simulink model "IEEE14_case"  (R2024b)
settings: Solver=FixedStepAuto  StartTime=0  StopTime=2  FixedStep=1e-7  RelTol=1e-3
values from neighbouring files (symbols this model uses):
  GFL_15_Bva = 0.009    [IEEE14_parameters.m]
  GFL_15_C_bus_pu = 7.179419    [IEEE14_parameters.m]
  GFL_15_f0 = 60    [IEEE14_parameters.m]
  GFL_15_I_id = 691.26967    [IEEE14_parameters.m]
  GFL_15_I_iq = 691.26967    [IEEE14_parameters.m]
  GFL_15_I_od = 45.2207    [IEEE14_parameters.m]
  GFL_15_I_oq = 45.2207    [IEEE14_parameters.m]
  GFL_15_I_pll = 0.78    [IEEE14_parameters.m]
  GFL_15_Kdi = 0.09    [IEEE14_parameters.m]
  GFL_15_Kdo = 0.9    [IEEE14_parameters.m]
  GFL_15_Kqi = 0.09    [IEEE14_parameters.m]
  GFL_15_Kqo = 0.9    [IEEE14_parameters.m]
  GFL_15_Lg_pu = 0.631447    [IEEE14_parameters.m]
  GFL_15_mode = 1    [IEEE14_parameters.m]
  GFL_15_P_id = 3.7166    [IEEE14_parameters.m]
  GFL_15_P_iq = 3.7166    [IEEE14_parameters.m]
  GFL_15_P_od = 0.4798    [IEEE14_parameters.m]
  GFL_15_P_oq = 0.4798    [IEEE14_parameters.m]
  GFL_15_P_pll = 290.42    [IEEE14_parameters.m]
  GFL_15_Qe_ref = 0.2    [IEEE14_parameters.m]
  GFL_15_Rg_pu = 0.024016    [IEEE14_parameters.m]
  GFL_15_Sbase = 1.000000e+4    (= 10000)    [IEEE14_parameters.m]
  GFL_15_Tdi = 0.01    [IEEE14_parameters.m]
  GFL_15_Tdo = 0.2    [IEEE14_parameters.m]
  GFL_15_Tqi = 0.01    [IEEE14_parameters.m]
  GFL_15_Tqo = 0.2    [IEEE14_parameters.m]
  GFL_15_Vbase = 380    [IEEE14_parameters.m]
  GFL_15_Vdc_ref = 1.011475    [IEEE14_parameters.m]
  GFL_15_Vdcbase = 700    [IEEE14_parameters.m]
  GFL_15_vq_ref = 0    [IEEE14_parameters.m]
  GFL_16_Bva = 0.002    [IEEE14_parameters.m]
  GFL_16_C_bus_pu = 7.179419    [IEEE14_parameters.m]
  GFL_16_f0 = 60    [IEEE14_parameters.m]
  GFL_16_I_id = 691.26967    [IEEE14_parameters.m]
  GFL_16_I_iq = 691.26967    [IEEE14_parameters.m]
  GFL_16_I_od = 45.2207    [IEEE14_parameters.m]
  GFL_16_I_oq = 45.2207    [IEEE14_parameters.m]
  GFL_16_I_pll = 0.78    [IEEE14_parameters.m]
  GFL_16_Kdi = 0.05    [IEEE14_parameters.m]
  GFL_16_Kdo = 0.5    [IEEE14_parameters.m]
  GFL_16_Kqi = 0.05    [IEEE14_parameters.m]
  GFL_16_Kqo = 0.5    [IEEE14_parameters.m]
  GFL_16_Lg_pu = 0.631447    [IEEE14_parameters.m]
  GFL_16_mode = 1    [IEEE14_parameters.m]
  GFL_16_P_id = 3.7166    [IEEE14_parameters.m]
  GFL_16_P_iq = 3.7166    [IEEE14_parameters.m]
  GFL_16_P_od = 0.4798    [IEEE14_parameters.m]
  GFL_16_P_oq = 0.4798    [IEEE14_parameters.m]
  GFL_16_P_pll = 290.42    [IEEE14_parameters.m]
  GFL_16_Qe_ref = 0.2    [IEEE14_parameters.m]
  GFL_16_Rg_pu = 0.024016    [IEEE14_parameters.m]
  GFL_16_Sbase = 1.000000e+4    (= 10000)    [IEEE14_parameters.m]
  GFL_16_Tdi = 0.01    [IEEE14_parameters.m]
  GFL_16_Tdo = 0.2    [IEEE14_parameters.m]
  GFL_16_Tqi = 0.01    [IEEE14_parameters.m]
  GFL_16_Tqo = 0.2    [IEEE14_parameters.m]
  GFL_16_Vbase = 380    [IEEE14_parameters.m]
  GFL_16_Vdc_ref = 1.01144    [IEEE14_parameters.m]
  GFL_16_Vdcbase = 700    [IEEE14_parameters.m]
  GFL_16_vq_ref = 0    [IEEE14_parameters.m]
  GFL_17_Bva = 0.002    [IEEE14_parameters.m]
  GFL_17_C_bus_pu = 7.179419    [IEEE14_parameters.m]
  GFL_17_f0 = 60    [IEEE14_parameters.m]
  GFL_17_I_id = 691.26967    [IEEE14_parameters.m]
  GFL_17_I_iq = 691.26967    [IEEE14_parameters.m]
  GFL_17_I_od = 45.2207    [IEEE14_parameters.m]
  GFL_17_I_oq = 45.2207    [IEEE14_parameters.m]
  GFL_17_I_pll = 0.78    [IEEE14_parameters.m]
  GFL_17_Kdi = 0.05    [IEEE14_parameters.m]
  GFL_17_Kdo = 0.5    [IEEE14_parameters.m]
  GFL_17_Kqi = 0.05    [IEEE14_parameters.m]
  GFL_17_Kqo = 0.5    [IEEE14_parameters.m]
  GFL_17_Lg_pu = 0.631447    [IEEE14_parameters.m]
  GFL_17_mode = 1    [IEEE14_parameters.m]
  GFL_17_P_id = 3.7166    [IEEE14_parameters.m]
  GFL_17_P_iq = 3.7166    [IEEE14_parameters.m]
  GFL_17_P_od = 0.4798    [IEEE14_parameters.m]
  GFL_17_P_oq = 0.4798    [IEEE14_parameters.m]
  GFL_17_P_pll = 290.42    [IEEE14_parameters.m]
  GFL_17_Qe_ref = 0.2    [IEEE14_parameters.m]
  GFL_17_Rg_pu = 0.024016    [IEEE14_parameters.m]
  GFL_17_Sbase = 1.000000e+4    (= 10000)    [IEEE14_parameters.m]
  GFL_17_Tdi = 0.01    [IEEE14_parameters.m]
  GFL_17_Tdo = 0.2    [IEEE14_parameters.m]
  GFL_17_Tqi = 0.01    [IEEE14_parameters.m]
  GFL_17_Tqo = 0.2    [IEEE14_parameters.m]
  GFL_17_Vbase = 380    [IEEE14_parameters.m]
  GFL_17_Vdc_ref = 1.011632    [IEEE14_parameters.m]
  GFL_17_Vdcbase = 700    [IEEE14_parameters.m]
  GFL_17_vq_ref = 0    [IEEE14_parameters.m]
  GFL_18_Bva = 0.002    [IEEE14_parameters.m]
  GFL_18_C_bus_pu = 7.179419    [IEEE14_parameters.m]
  GFL_18_f0 = 60    [IEEE14_parameters.m]
  GFL_18_I_id = 691.26967    [IEEE14_parameters.m]
  GFL_18_I_iq = 691.26967    [IEEE14_parameters.m]
  GFL_18_I_od = 45.2207    [IEEE14_parameters.m]
  GFL_18_I_oq = 45.2207    [IEEE14_parameters.m]
  GFL_18_I_pll = 0.78    [IEEE14_parameters.m]
  GFL_18_Kdi = 0.05    [IEEE14_parameters.m]
  GFL_18_Kdo = 0.5    [IEEE14_parameters.m]
  GFL_18_Kqi = 0.05    [IEEE14_parameters.m]
  GFL_18_Kqo = 0.5    [IEEE14_parameters.m]
  GFL_18_Lg_pu = 0.631447    [IEEE14_parameters.m]
  GFL_18_mode = 1    [IEEE14_parameters.m]
  GFL_18_P_id = 3.7166    [IEEE14_parameters.m]
  GFL_18_P_iq = 3.7166    [IEEE14_parameters.m]
  GFL_18_P_od = 0.4798    [IEEE14_parameters.m]
  GFL_18_P_oq = 0.4798    [IEEE14_parameters.m]
  GFL_18_P_pll = 290.42    [IEEE14_parameters.m]
  GFL_18_Qe_ref = 0.2    [IEEE14_parameters.m]
  GFL_18_Rg_pu = 0.024016    [IEEE14_parameters.m]
  GFL_18_Sbase = 1.000000e+4    (= 10000)    [IEEE14_parameters.m]
  GFL_18_Tdi = 0.01    [IEEE14_parameters.m]
  GFL_18_Tdo = 0.2    [IEEE14_parameters.m]
  GFL_18_Tqi = 0.01    [IEEE14_parameters.m]
  GFL_18_Tqo = 0.2    [IEEE14_parameters.m]
  GFL_18_Vbase = 380    [IEEE14_parameters.m]
  GFL_18_Vdc_ref = 1.011572    [IEEE14_parameters.m]
  GFL_18_Vdcbase = 700    [IEEE14_parameters.m]
  GFL_18_vq_ref = 0    [IEEE14_parameters.m]
  ... (+180 more)
(part 12 of 25)

== system IEEE14_case/GFL_16/d_i_gq_GFL_16_block ==
  note: d_i_gq_GFL_16 in case14gfl
      | $\frac{2\,\pi \,\mathrm{Sbase}\,f_{0}\,\left(\Phi _{\mathrm{gd},\mathrm{GFL},16}+P_{\mathrm{iq}}\,\left(\mathrm{Iqv}_{\mathrm{GFL},16}+\Phi _{\mathrm{gc},\mathrm{GFL},16}-i_{\mathrm{gq},\mathrm{GFL},16}-P_{\mathrm{oq}}\,\left(\mathrm{Qe}_{\mathrm{ref}}\,\mathrm{Sbase}+1.73205080756888\,\mathrm{Vbase}\,i_{\mathrm{gd},\mathrm{GFL},16}\,\left(v_{q,\mathrm{GFL},16}\,\cos\left(\theta _{\mathrm{pll},\mathrm{GFL},16}\right)+v_{d,\mathrm{GFL},16}\,\sin\left(\theta _{\mathrm{pll},\mathrm{GFL},16}\right)\right)+1.73205080756888\,\mathrm{Vbase}\,i_{\mathrm{gq},\mathrm{GFL},16}\,\left(v_{d,\mathrm{GFL},16}\,\cos\left(\theta _{\mathrm{pll},\mathrm{GFL},16}\right)-v_{q,\mathrm{GFL},16}\,\sin\left(\theta _{\mathrm{pll},\mathrm{GFL},16}\right)\right)\right)+\mathrm{Bva}\,\mathrm{Vbase}\,\left(v_{q,\mathrm{GFL},16}\,\cos\left(\theta _{\mathrm{pll},\mathrm{GFL},16}\right)+v_{d,\mathrm{GFL},16}\,\sin\left(\theta _{\mathrm{pll},\mathrm{GFL},16}\right)\right)\right)-\frac{\mathrm{Rg}_{\mathrm{pu}}\,{\mathrm{Vbase}}^2\,i_{\mathrm{gq},\mathrm{GFL},16}}{\mathrm{Sbase}}\right)}{\mathrm{Lg}_{\mathrm{pu}}\,{\mathrm{Vbase}}^2}$
      | Automatically generated on 2025-10-09 21:35:48 .
  Input_v_d_GFL_16_26005 : Inport
  State_theta_pll_GFL_16_b9b0c : Inport  Port=2
  Input_v_q_GFL_16_f5e00 : Inport  Port=3
  State_theta_pll_GFL_16_3325f : Inport  Port=4
  State_Iqv_GFL_16_fce4f : Inport  Port=5
  State_i_gd_GFL_16_461cd : Inport  Port=6
  Input_v_d_GFL_16_21396 : Inport  Port=7
  State_theta_pll_GFL_16_b6938 : Inport  Port=8
  Input_v_q_GFL_16_5c00e : Inport  Port=9
  State_theta_pll_GFL_16_ce5b5 : Inport  Port=10
  State_i_gq_GFL_16_8af0d : Inport  Port=11
  Input_v_d_GFL_16_f3aaf : Inport  Port=12
  State_theta_pll_GFL_16_f68d0 : Inport  Port=13
  Input_v_q_GFL_16_4d2d7 : Inport  Port=14
  State_theta_pll_GFL_16_2ae3b : Inport  Port=15
  State_Phi_gc_GFL_16_ded18 : Inport  Port=16
  State_i_gq_GFL_16_f0d16 : Inport  Port=17
  State_Phi_gd_GFL_16_6ff49 : Inport  Port=18
  State_i_gq_GFL_16_bb299 : Inport  Port=19
  Add_1f236 : Sum
  Add_902ad : Sum
  Add_90e5e : Sum
  Add_b2698 : Sum
  Add_d010b : Sum
  Add_ed010 : Sum
  Constant_-1_4b2a3 : Constant  Value=-1
  Constant_1.73205080756888_41091 : Constant  Value=1.73205080756888
  Constant_1.73205080756888_fcb3e : Constant  Value=1.73205080756888
  Constant_2.0_22626 : Constant  Value=2.0
  Constant_2.0_38ada : Constant  Value=2.0
  Constant_2.0_a6037 : Constant  Value=2.0
  Constant_Bva_7a2f5 : Constant  Value=Bva
  Constant_Lg_pu_7f2f3 : Constant  Value=Lg_pu
  Constant_P_iq_ae706 : Constant  Value=P_iq
  Constant_P_oq_d800d : Constant  Value=P_oq
  Constant_Qe_ref_48f82 : Constant  Value=Qe_ref
  Constant_Rg_pu_1fb6c : Constant  Value=Rg_pu
  Constant_Sbase_2a5f4 : Constant  Value=Sbase
  Constant_Sbase_8d4df : Constant  Value=Sbase
  Constant_Sbase_d2429 : Constant  Value=Sbase
  Constant_Vbase_52c7c : Constant  Value=Vbase
  Constant_Vbase_77d71 : Constant  Value=Vbase
  Constant_Vbase_9d288 : Constant  Value=Vbase
  Constant_Vbase_cc3fd : Constant  Value=Vbase
  Constant_Vbase_f36e9 : Constant  Value=Vbase
  Constant_f0_15919 : Constant  Value=f0
  Constant_pi_ae5c5 : Constant  Value=pi
  Divide_358c2 : Product  Inputs=*/
  Divide_d98bc : Product  Inputs=*/
  MathFunc_cos_1f83c : Trigonometry  Operator=cos
  MathFunc_cos_2f6c0 : Trigonometry  Operator=cos
  MathFunc_cos_612b0 : Trigonometry  Operator=cos
  MathFunc_sin_4af8b : Trigonometry
  MathFunc_sin_9c669 : Trigonometry
  MathFunc_sin_cb3b8 : Trigonometry
  Power_64a0d : Math  Operator=pow
  Power_c9ffe : Math  Operator=pow
  Product_0ecab : Product
  Product_0f8e8 : Product
  Product_125e1 : Product
  Product_2253b : Product
  Product_24ac4 : Product
  Product_3d9b9 : Product
  Product_45584 : Product
  Product_5de20 : Product
  Product_630cf : Product
  Product_76e52 : Product
  Product_7ef05 : Product
  Product_7fa9f : Product
  Product_93679 : Product
  Product_95eb5 : Product
  Product_96ca3 : Product
  Product_9f0a3 : Product
  Product_a28aa : Product
  Product_a51bb : Product
  Product_c0fca : Product
  Product_d9703 : Product
  Product_e0f5e : Product
  Product_e1d29 : Product
  Product_f68a2 : Product
  Product_fdb7e : Product
  Product_ffb6f : Product
  Subtract_3c982 : Sum  Inputs=+-
  Subtract_9e73c : Sum  Inputs=+-
  Subtract_aaa71 : Sum  Inputs=+-
  Subtract_dcd4c : Sum  Inputs=+-
  Subtract_f9644 : Sum  Inputs=+-
  Blockout_d_i_gq_GFL_16_4ea9b : Outport
  wires:
  State_theta_pll_GFL_16_b6938/1 -> MathFunc_sin_9c669/1
  MathFunc_sin_9c669/1 -> Product_93679/2
  Subtract_f9644/1 -> Product_e1d29/2
  Constant_Vbase_f36e9/1 -> Product_c0fca/2
  State_theta_pll_GFL_16_ce5b5/1 -> MathFunc_cos_2f6c0/1
  MathFunc_cos_2f6c0/1 -> Product_9f0a3/2
  Product_c0fca/1 -> Product_fdb7e/1
  Constant_1.73205080756888_41091/1 -> Product_c0fca/1
  Product_93679/1 -> Add_d010b/1
  Input_v_d_GFL_16_21396/1 -> Product_93679/1
  Input_v_q_GFL_16_5c00e/1 -> Product_9f0a3/1
  Constant_Sbase_d2429/1 -> Product_5de20/2
  MathFunc_cos_612b0/1 -> Product_96ca3/2
  State_Phi_gd_GFL_16_6ff49/1 -> Add_ed010/2
  State_theta_pll_GFL_16_f68d0/1 -> MathFunc_cos_612b0/1
  Product_9f0a3/1 -> Add_d010b/2
  Constant_Sbase_8d4df/1 -> Divide_358c2/2
  State_theta_pll_GFL_16_2ae3b/1 -> MathFunc_sin_4af8b/1
  MathFunc_sin_cb3b8/1 -> Product_0f8e8/2
  State_theta_pll_GFL_16_b9b0c/1 -> MathFunc_sin_cb3b8/1
  State_theta_pll_GFL_16_3325f/1 -> MathFunc_cos_1f83c/1
  Constant_-1_4b2a3/1 -> Product_ffb6f/1
  Constant_Qe_ref_48f82/1 -> Product_ffb6f/2
  Constant_1.73205080756888_fcb3e/1 -> Product_a51bb/1
  State_i_gd_GFL_16_461cd/1 -> Product_fdb7e/2
  Constant_Vbase_52c7c/1 -> Power_c9ffe/1
  Product_3d9b9/1 -> Add_1f236/1
  Constant_Vbase_cc3fd/1 -> Product_a51bb/2
  State_i_gq_GFL_16_f0d16/1 -> Subtract_9e73c/2
  Input_v_d_GFL_16_f3aaf/1 -> Product_96ca3/1
  Input_v_q_GFL_16_4d2d7/1 -> Product_a28aa/1
  Constant_2.0_22626/1 -> Product_7ef05/1
  MathFunc_sin_4af8b/1 -> Product_a28aa/2
  Product_a28aa/1 -> Subtract_dcd4c/2
  Input_v_d_GFL_16_26005/1 -> Product_0f8e8/1
  Input_v_q_GFL_16_f5e00/1 -> Product_7fa9f/1
  Subtract_dcd4c/1 -> Product_e0f5e/2
  MathFunc_cos_1f83c/1 -> Product_7fa9f/2
  Product_ffb6f/1 -> Product_5de20/1
  Product_fdb7e/1 -> Product_d9703/1
  Add_d010b/1 -> Product_d9703/2
  Add_90e5e/1 -> Subtract_9e73c/1
  Product_a51bb/1 -> Product_630cf/1
  State_i_gq_GFL_16_8af0d/1 -> Product_630cf/2
  Product_96ca3/1 -> Subtract_dcd4c/1
  Constant_Bva_7a2f5/1 -> Product_2253b/1
  Constant_pi_ae5c5/1 -> Product_7ef05/2
  Constant_Vbase_9d288/1 -> Product_2253b/2
  Product_0f8e8/1 -> Add_902ad/1
  Product_7fa9f/1 -> Add_902ad/2
  Subtract_9e73c/1 -> Product_24ac4/2
  Product_5de20/1 -> Subtract_aaa71/1
  Constant_Vbase_77d71/1 -> Power_64a0d/1
  Product_d9703/1 -> Subtract_aaa71/2
  Product_630cf/1 -> Product_e0f5e/1
  Power_c9ffe/1 -> Product_f68a2/2
  Product_2253b/1 -> Product_3d9b9/1
  Constant_Sbase_2a5f4/1 -> Product_45584/2
  Add_902ad/1 -> Product_3d9b9/2
  Subtract_aaa71/1 -> Subtract_f9644/1
  Product_e0f5e/1 -> Subtract_f9644/2
  State_Iqv_GFL_16_fce4f/1 -> Add_1f236/2
  Constant_P_oq_d800d/1 -> Product_e1d29/1
  Add_1f236/1 -> Add_b2698/1
  Product_e1d29/1 -> Add_b2698/2
  Add_b2698/1 -> Add_90e5e/1
  State_Phi_gc_GFL_16_ded18/1 -> Add_90e5e/2
  Constant_2.0_a6037/1 -> Power_c9ffe/2
  Constant_Rg_pu_1fb6c/1 -> Product_f68a2/1
  Constant_P_iq_ae706/1 -> Product_24ac4/1
  Product_f68a2/1 -> Product_0ecab/1
  State_i_gq_GFL_16_bb299/1 -> Product_0ecab/2
  Product_7ef05/1 -> Product_45584/1
  Product_24ac4/1 -> Add_ed010/1
  Product_0ecab/1 -> Divide_358c2/1
  Product_45584/1 -> Product_76e52/1
  Constant_f0_15919/1 -> Product_76e52/2
  Add_ed010/1 -> Subtract_3c982/1
  Divide_358c2/1 -> Subtract_3c982/2
  Constant_2.0_38ada/1 -> Power_64a0d/2
  Product_76e52/1 -> Product_95eb5/1
  Subtract_3c982/1 -> Product_95eb5/2
  Constant_Lg_pu_7f2f3/1 -> Product_125e1/1
  Power_64a0d/1 -> Product_125e1/2
  Product_95eb5/1 -> Divide_d98bc/1
  Product_125e1/1 -> Divide_d98bc/2
  Divide_d98bc/1 -> Blockout_d_i_gq_GFL_16_4ea9b/1

== system IEEE14_case/GFL_16/d_theta_pll_GFL_16_block ==
  note: d_theta_pll_GFL_16 in case14gfl
      | $\mathrm{Phipll}_{\mathrm{GFL},16}-P_{\mathrm{pll}}\,\left(\mathrm{vq}_{\mathrm{ref}}+v_{q,\mathrm{GFL},16}\,\cos\left(\theta _{\mathrm{pll},\mathrm{GFL},16}\right)+v_{d,\mathrm{GFL},16}\,\sin\left(\theta _{\mathrm{pll},\mathrm{GFL},16}\right)\right)$
      | Automatically generated on 2025-10-09 21:36:05 .
  Input_v_d_GFL_16_c3931 : Inport
  State_theta_pll_GFL_16_60b13 : Inport  Port=2
  Input_v_q_GFL_16_f8c47 : Inport  Port=3
  State_theta_pll_GFL_16_eb390 : Inport  Port=4
  State_Phipll_GFL_16_9e2b9 : Inport  Port=5
  Add_7626c : Sum
  Constant_-1_d55e9 : Constant  Value=-1
  Constant_P_pll_b3652 : Constant  Value=P_pll
  Constant_vq_ref_9ec67 : Constant  Value=vq_ref
  MathFunc_cos_68f81 : Trigonometry  Operator=cos
  MathFunc_sin_003f3 : Trigonometry
  Product_2e053 : Product
  Product_35cda : Product
  Product_c0d6e : Product
  Product_c6d12 : Product
  Subtract_48f00 : Sum  Inputs=+-
  Subtract_4de10 : Sum  Inputs=+-
  Blockout_d_theta_pll_GFL_16_374a4 : Outport
  wires:
  Constant_vq_ref_9ec67/1 -> Subtract_4de10/2
  MathFunc_cos_68f81/1 -> Product_c0d6e/2
  Product_2e053/1 -> Product_c6d12/1
  Constant_-1_d55e9/1 -> Product_2e053/1
  Input_v_d_GFL_16_c3931/1 -> Product_2e053/2
  State_theta_pll_GFL_16_60b13/1 -> MathFunc_sin_003f3/1
  State_theta_pll_GFL_16_eb390/1 -> MathFunc_cos_68f81/1
  MathFunc_sin_003f3/1 -> Product_c6d12/2
  Input_v_q_GFL_16_f8c47/1 -> Product_c0d6e/1
  Product_c6d12/1 -> Subtract_48f00/1
  Product_c0d6e/1 -> Subtract_48f00/2
  Subtract_48f00/1 -> Subtract_4de10/1
  Constant_P_pll_b3652/1 -> Product_35cda/1
  Subtract_4de10/1 -> Product_35cda/2
  Product_35cda/1 -> Add_7626c/1
  State_Phipll_GFL_16_9e2b9/1 -> Add_7626c/2
  Add_7626c/1 -> Blockout_d_theta_pll_GFL_16_374a4/1

== system IEEE14_case/GFL_16/e_dc_GFL_16_block ==
  note: e_dc_GFL_16 in case14gfl
      | $\frac{V_{\mathrm{dc},\mathrm{GFL},16}}{\mathrm{Vdcbase}}$
      | Automatically generated on 2025-10-09 21:36:23 .
  State_V_dc_GFL_16_ba6ae : Inport
  Constant_Vdcbase_fd435 : Constant  Value=Vdcbase
  Divide_18da4 : Product  Inputs=*/
  Blockout_e_dc_GFL_16_30897 : Outport
  wires:
  State_V_dc_GFL_16_ba6ae/1 -> Divide_18da4/1
  Constant_Vdcbase_fd435/1 -> Divide_18da4/2
  Divide_18da4/1 -> Blockout_e_dc_GFL_16_30897/1

== system IEEE14_case/GFL_16/i_d_GFL_16_block ==
  note: i_d_GFL_16 in case14gfl
      | $0.00658179306876173\,i_{\mathrm{gd},\mathrm{GFL},16}\,\cos\left(\theta _{\mathrm{pll},\mathrm{GFL},16}\right)+0.00658179306876173\,i_{\mathrm{gq},\mathrm{GFL},16}\,\sin\left(\theta _{\mathrm{pll},\mathrm{GFL},16}\right)$
      | Automatically generated on 2025-10-09 21:36:22 .
  State_i_gd_GFL_16_f9181 : Inport
  State_theta_pll_GFL_16_be048 : Inport  Port=2
  State_i_gq_GFL_16_5d9af : Inport  Port=3
  State_theta_pll_GFL_16_4b91a : Inport  Port=4
  Add_e2555 : Sum
  Constant_0.00658179306876173_ae954 : Constant  Value=0.00658179306876173
  Constant_0.00658179306876173_b6366 : Constant  Value=0.00658179306876173
  MathFunc_cos_8767b : Trigonometry  Operator=cos
  MathFunc_sin_49c71 : Trigonometry
  Product_74789 : Product
  Product_a340e : Product
  Product_b858c : Product
  Product_e5950 : Product
  Blockout_i_d_GFL_16_cb76b : Outport
  wires:
  Constant_0.00658179306876173_ae954/1 -> Product_74789/1
  State_i_gd_GFL_16_f9181/1 -> Product_74789/2
  Constant_0.00658179306876173_b6366/1 -> Product_a340e/1
  Product_74789/1 -> Product_e5950/1
  State_theta_pll_GFL_16_be048/1 -> MathFunc_cos_8767b/1
  MathFunc_sin_49c71/1 -> Product_b858c/2
  State_theta_pll_GFL_16_4b91a/1 -> MathFunc_sin_49c71/1
  State_i_gq_GFL_16_5d9af/1 -> Product_a340e/2
  MathFunc_cos_8767b/1 -> Product_e5950/2
  Product_a340e/1 -> Product_b858c/1
  Product_e5950/1 -> Add_e2555/1
  Product_b858c/1 -> Add_e2555/2
  Add_e2555/1 -> Blockout_i_d_GFL_16_cb76b/1

== system IEEE14_case/GFL_16/i_q_GFL_16_block ==
  note: i_q_GFL_16 in case14gfl
      | $0.00658179306876173\,i_{\mathrm{gq},\mathrm{GFL},16}\,\cos\left(\theta _{\mathrm{pll},\mathrm{GFL},16}\right)-0.00658179306876173\,i_{\mathrm{gd},\mathrm{GFL},16}\,\sin\left(\theta _{\mathrm{pll},\mathrm{GFL},16}\right)$
      | Automatically generated on 2025-10-09 21:36:23 .
  State_i_gd_GFL_16_ab236 : Inport
  State_theta_pll_GFL_16_38575 : Inport  Port=2
  State_i_gq_GFL_16_367d1 : Inport  Port=3
  State_theta_pll_GFL_16_9c98e : Inport  Port=4
  Add_02676 : Sum
  Constant_-0.00658179306876173_48262 : Constant  Value=-0.00658179306876173
  Constant_0.00658179306876173_3e7d2 : Constant  Value=0.00658179306876173
  MathFunc_cos_cb348 : Trigonometry  Operator=cos
  MathFunc_sin_a77fd : Trigonometry
  Product_1db57 : Product
  Product_29a7e : Product
  Product_6d2ca : Product
  Product_a6e96 : Product
  Blockout_i_q_GFL_16_30f67 : Outport
  wires:
  State_theta_pll_GFL_16_38575/1 -> MathFunc_sin_a77fd/1
  MathFunc_sin_a77fd/1 -> Product_a6e96/2
  Constant_-0.00658179306876173_48262/1 -> Product_6d2ca/1
  State_i_gd_GFL_16_ab236/1 -> Product_6d2ca/2
  Constant_0.00658179306876173_3e7d2/1 -> Product_29a7e/1
  State_theta_pll_GFL_16_9c98e/1 -> MathFunc_cos_cb348/1
  State_i_gq_GFL_16_367d1/1 -> Product_29a7e/2
  Product_29a7e/1 -> Product_1db57/1
  Product_6d2ca/1 -> Product_a6e96/1
  MathFunc_cos_cb348/1 -> Product_1db57/2
  Product_a6e96/1 -> Add_02676/1
  Product_1db57/1 -> Add_02676/2
  Add_02676/1 -> Blockout_i_q_GFL_16_30f67/1

== system IEEE14_case/GFL_17/d_Idv_GFL_17_block ==
  note: d_Idv_GFL_17 in case14gfl
      | $-\frac{\mathrm{Idv}_{\mathrm{GFL},17}+\mathrm{Kdo}\,\left(\mathrm{Vbase}\,\left(v_{q,\mathrm{GFL},17}\,\cos\left(\theta _{\mathrm{pll},\mathrm{GFL},17}\right)+v_{d,\mathrm{GFL},17}\,\sin\left(\theta _{\mathrm{pll},\mathrm{GFL},17}\right)\right)+\frac{\Psi _{d,\mathrm{GFL},17}+\mathrm{Kdi}\,\mathrm{Vbase}\,\left(v_{q,\mathrm{GFL},17}\,\cos\left(\theta _{\mathrm{pll},\mathrm{GFL},17}\right)+v_{d,\mathrm{GFL},17}\,\sin\left(\theta _{\mathrm{pll},\mathrm{GFL},17}\right)\right)}{\mathrm{Tdi}}\right)}{\mathrm{Tdo}}$
      | Automatically generated on 2025-10-09 21:37:09 .
  State_Idv_GFL_17_dbb4f : Inport
  Input_v_d_GFL_17_0e53b : Inport  Port=2
  State_theta_pll_GFL_17_9e194 : Inport  Port=3
  Input_v_q_GFL_17_e3e51 : Inport  Port=4
  State_theta_pll_GFL_17_44aa2 : Inport  Port=5
  Input_v_d_GFL_17_235ef : Inport  Port=6
  State_theta_pll_GFL_17_82810 : Inport  Port=7
  Input_v_q_GFL_17_30fdf : Inport  Port=8
  State_theta_pll_GFL_17_629fa : Inport  Port=9
  State_Psi_d_GFL_17_f48a9 : Inport  Port=10
  Add_19e0d : Sum
  Add_407e1 : Sum
  Add_9e12e : Sum
  Add_e059e : Sum
  Constant_-1_60b73 : Constant  Value=-1
  Constant_-1_6492a : Constant  Value=-1
  Constant_-1_7eaa5 : Constant  Value=-1
  Constant_Kdi_1c444 : Constant  Value=Kdi
  Constant_Kdo_3c9a4 : Constant  Value=Kdo
  Constant_Tdi_7b760 : Constant  Value=Tdi
  Constant_Tdo_79e16 : Constant  Value=Tdo
  Constant_Vbase_3644b : Constant  Value=Vbase
  Constant_Vbase_fb71e : Constant  Value=Vbase
  Divide_7e80e : Product  Inputs=*/
  Divide_8f2a2 : Product  Inputs=*/
  MathFunc_cos_0a357 : Trigonometry  Operator=cos
  MathFunc_cos_f652e : Trigonometry  Operator=cos
  MathFunc_sin_70d65 : Trigonometry
  MathFunc_sin_a2488 : Trigonometry
  Product_2f4b2 : Product
  Product_5021f : Product
  Product_54b19 : Product
  Product_56195 : Product
  Product_68e02 : Product
  Product_76722 : Product
  Product_8e4b6 : Product
  Product_ab766 : Product
  Product_b5de5 : Product
  Product_d24d6 : Product
  Product_e8be3 : Product
  Subtract_1449a : Sum  Inputs=+-
  Blockout_d_Idv_GFL_17_3c079 : Outport
  wires:
  Product_2f4b2/1 -> Add_9e12e/2
  Input_v_q_GFL_17_e3e51/1 -> Product_2f4b2/1
  MathFunc_cos_0a357/1 -> Product_d24d6/2
  Product_68e02/1 -> Product_5021f/1
  Constant_Kdi_1c444/1 -> Product_ab766/2
  Constant_Tdo_79e16/1 -> Divide_8f2a2/2
  State_theta_pll_GFL_17_82810/1 -> MathFunc_sin_70d65/1
  Add_407e1/1 -> Divide_8f2a2/1
  MathFunc_sin_70d65/1 -> Product_8e4b6/2
  State_theta_pll_GFL_17_629fa/1 -> MathFunc_cos_0a357/1
  Constant_Vbase_fb71e/1 -> Product_68e02/2
  Product_ab766/1 -> Product_68e02/1
  Constant_-1_60b73/1 -> Product_ab766/1
  Input_v_d_GFL_17_235ef/1 -> Product_8e4b6/1
  Product_d24d6/1 -> Add_19e0d/2
  Input_v_q_GFL_17_30fdf/1 -> Product_d24d6/1
  State_theta_pll_GFL_17_9e194/1 -> MathFunc_sin_a2488/1
  Constant_Tdi_7b760/1 -> Divide_7e80e/2
  MathFunc_cos_f652e/1 -> Product_2f4b2/2
  State_theta_pll_GFL_17_44aa2/1 -> MathFunc_cos_f652e/1
  Product_8e4b6/1 -> Add_19e0d/1
  Product_76722/1 -> Add_9e12e/1
  Input_v_d_GFL_17_0e53b/1 -> Product_76722/1
  MathFunc_sin_a2488/1 -> Product_76722/2
  Add_19e0d/1 -> Product_5021f/2
  Product_54b19/1 -> Product_56195/1
  Constant_-1_6492a/1 -> Product_54b19/1
  Add_9e12e/1 -> Product_56195/2
  Constant_Vbase_3644b/1 -> Product_54b19/2
  Product_5021f/1 -> Subtract_1449a/1
  State_Psi_d_GFL_17_f48a9/1 -> Subtract_1449a/2
  Subtract_1449a/1 -> Divide_7e80e/1
  Product_56195/1 -> Add_e059e/1
  Divide_7e80e/1 -> Add_e059e/2
  Constant_-1_7eaa5/1 -> Product_e8be3/1
  State_Idv_GFL_17_dbb4f/1 -> Product_e8be3/2
  Constant_Kdo_3c9a4/1 -> Product_b5de5/1
  Add_e059e/1 -> Product_b5de5/2
  Product_e8be3/1 -> Add_407e1/1
  Product_b5de5/1 -> Add_407e1/2
  Divide_8f2a2/1 -> Blockout_d_Idv_GFL_17_3c079/1

== system IEEE14_case/GFL_17/d_Iqv_GFL_17_block ==
  note: d_Iqv_GFL_17 in case14gfl
      | $-\frac{\mathrm{Iqv}_{\mathrm{GFL},17}-\mathrm{Kqo}\,\left(\mathrm{Vbase}\,\left(v_{d,\mathrm{GFL},17}\,\cos\left(\theta _{\mathrm{pll},\mathrm{GFL},17}\right)-v_{q,\mathrm{GFL},17}\,\sin\left(\theta _{\mathrm{pll},\mathrm{GFL},17}\right)\right)-\frac{\Psi _{q,\mathrm{GFL},17}-\mathrm{Kqi}\,\mathrm{Vbase}\,\left(v_{d,\mathrm{GFL},17}\,\cos\left(\theta _{\mathrm{pll},\mathrm{GFL},17}\right)-v_{q,\mathrm{GFL},17}\,\sin\left(\theta _{\mathrm{pll},\mathrm{GFL},17}\right)\right)}{\mathrm{Tqi}}\right)}{\mathrm{Tqo}}$
      | Automatically generated on 2025-10-09 21:37:11 .
  State_Iqv_GFL_17_66272 : Inport
  Input_v_d_GFL_17_2ae22 : Inport  Port=2
  State_theta_pll_GFL_17_38143 : Inport  Port=3
  Input_v_q_GFL_17_45d80 : Inport  Port=4
  State_theta_pll_GFL_17_2973d : Inport  Port=5
  Input_v_d_GFL_17_ad61a : Inport  Port=6
  State_theta_pll_GFL_17_aa9de : Inport  Port=7
  Input_v_q_GFL_17_37f0a : Inport  Port=8
  State_theta_pll_GFL_17_b5422 : Inport  Port=9
  State_Psi_q_GFL_17_98c01 : Inport  Port=10
  Add_c0ed2 : Sum
  Add_e9412 : Sum
  Constant_-1_a3351 : Constant  Value=-1
  Constant_Kqi_10364 : Constant  Value=Kqi
  Constant_Kqo_8d5df : Constant  Value=Kqo
  Constant_Tqi_7501f : Constant  Value=Tqi
  Constant_Tqo_f9a2c : Constant  Value=Tqo
  Constant_Vbase_32ff6 : Constant  Value=Vbase
  Constant_Vbase_cc720 : Constant  Value=Vbase
  Divide_0e743 : Product  Inputs=*/
  Divide_b6944 : Product  Inputs=*/
  MathFunc_cos_576a1 : Trigonometry  Operator=cos
  MathFunc_cos_7bffe : Trigonometry  Operator=cos
  MathFunc_sin_54d42 : Trigonometry
  MathFunc_sin_abdec : Trigonometry
  Product_1c4f8 : Product
  Product_26ece : Product
  Product_96666 : Product
  Product_99464 : Product
  Product_9a84c : Product
  Product_9ab5c : Product
  Product_c00e0 : Product
  Product_c76d0 : Product
  Product_ce9ff : Product
  Subtract_3e13e : Sum  Inputs=+-
  Subtract_5d400 : Sum  Inputs=+-
  Subtract_a6b1b : Sum  Inputs=+-
  Blockout_d_Iqv_GFL_17_0648b : Outport
  wires:
  Constant_Tqo_f9a2c/1 -> Divide_0e743/2
  State_theta_pll_GFL_17_aa9de/1 -> MathFunc_cos_576a1/1
  MathFunc_cos_576a1/1 -> Product_c00e0/2
  State_theta_pll_GFL_17_2973d/1 -> MathFunc_sin_54d42/1
  State_theta_pll_GFL_17_b5422/1 -> MathFunc_sin_abdec/1
  Input_v_d_GFL_17_ad61a/1 -> Product_c00e0/1
  Add_c0ed2/1 -> Product_c76d0/2
  Input_v_q_GFL_17_37f0a/1 -> Product_99464/1
  MathFunc_sin_abdec/1 -> Product_99464/2
  Constant_Kqo_8d5df/1 -> Product_c76d0/1
  State_theta_pll_GFL_17_38143/1 -> MathFunc_cos_7bffe/1
  Constant_Kqi_10364/1 -> Product_ce9ff/1
  Constant_Vbase_32ff6/1 -> Product_ce9ff/2
  Product_c00e0/1 -> Subtract_5d400/1
  Product_99464/1 -> Subtract_5d400/2
  Input_v_d_GFL_17_2ae22/1 -> Product_9ab5c/1
  MathFunc_cos_7bffe/1 -> Product_9ab5c/2
  Add_e9412/1 -> Divide_0e743/1
  Product_26ece/1 -> Subtract_a6b1b/2
  Input_v_q_GFL_17_45d80/1 -> Product_26ece/1
  MathFunc_sin_54d42/1 -> Product_26ece/2
  Divide_0e743/1 -> Blockout_d_Iqv_GFL_17_0648b/1
  Product_ce9ff/1 -> Product_9a84c/1
  Subtract_5d400/1 -> Product_9a84c/2
  Product_9ab5c/1 -> Subtract_a6b1b/1
  Product_9a84c/1 -> Subtract_3e13e/1
  State_Psi_q_GFL_17_98c01/1 -> Subtract_3e13e/2
  Constant_Vbase_cc720/1 -> Product_96666/1
  Subtract_a6b1b/1 -> Product_96666/2
  Subtract_3e13e/1 -> Divide_b6944/1
  Constant_Tqi_7501f/1 -> Divide_b6944/2
  Product_96666/1 -> Add_c0ed2/1
  Divide_b6944/1 -> Add_c0ed2/2
  Constant_-1_a3351/1 -> Product_1c4f8/1
  State_Iqv_GFL_17_66272/1 -> Product_1c4f8/2
  Product_1c4f8/1 -> Add_e9412/1
  Product_c76d0/1 -> Add_e9412/2

== system IEEE14_case/GFL_17/d_Phi_ga_GFL_17_block ==
  note: d_Phi_ga_GFL_17 in case14gfl
      | $I_{\mathrm{od}}\,\left(V_{\mathrm{dc},\mathrm{GFL},17}-\mathrm{Vdcbase}\,\mathrm{Vdc}_{\mathrm{ref}}\right)$
      | Automatically generated on 2025-10-09 21:36:57 .
  State_V_dc_GFL_17_b46a6 : Inport
  Constant_I_od_b3062 : Constant  Value=I_od
  Constant_Vdc_ref_d7bbc : Constant  Value=Vdc_ref
  Constant_Vdcbase_d5ce1 : Constant  Value=Vdcbase
  Product_326a8 : Product
  Product_7ada9 : Product
  Subtract_ba96c : Sum  Inputs=+-
  Blockout_d_Phi_ga_GFL_17_7246c : Outport
  wires:
  Constant_Vdc_ref_d7bbc/1 -> Product_7ada9/1
  State_V_dc_GFL_17_b46a6/1 -> Subtract_ba96c/1
  Constant_Vdcbase_d5ce1/1 -> Product_7ada9/2
  Product_7ada9/1 -> Subtract_ba96c/2
  Subtract_ba96c/1 -> Product_326a8/2
  Constant_I_od_b3062/1 -> Product_326a8/1
  Product_326a8/1 -> Blockout_d_Phi_ga_GFL_17_7246c/1

== system IEEE14_case/GFL_17/d_Phi_gb_GFL_17_block ==
  note: d_Phi_gb_GFL_17 in case14gfl
      | $I_{\mathrm{id}}\,\left(\mathrm{Idv}_{\mathrm{GFL},17}+\Phi _{\mathrm{ga},\mathrm{GFL},17}-i_{\mathrm{gd},\mathrm{GFL},17}+P_{\mathrm{od}}\,\left(V_{\mathrm{dc},\mathrm{GFL},17}-\mathrm{Vdcbase}\,\mathrm{Vdc}_{\mathrm{ref}}\right)-\mathrm{Bva}\,\mathrm{Vbase}\,\left(v_{d,\mathrm{GFL},17}\,\cos\left(\theta _{\mathrm{pll},\mathrm{GFL},17}\right)-v_{q,\mathrm{GFL},17}\,\sin\left(\theta _{\mathrm{pll},\mathrm{GFL},17}\right)\right)\right)$
      | Automatically generated on 2025-10-09 21:36:59 .
  Input_v_d_GFL_17_375e3 : Inport
  State_theta_pll_GFL_17_d7184 : Inport  Port=2
  Input_v_q_GFL_17_c3fa8 : Inport  Port=3
  State_theta_pll_GFL_17_d1250 : Inport  Port=4
  State_Idv_GFL_17_5ec1c : Inport  Port=5
  State_V_dc_GFL_17_71b96 : Inport  Port=6
  State_Phi_ga_GFL_17_0e94a : Inport  Port=7
  State_i_gd_GFL_17_f44e4 : Inport  Port=8
  Add_0e360 : Sum
  Add_62c7f : Sum
  Add_c91bc : Sum
  Constant_-1_b59c1 : Constant  Value=-1
  Constant_Bva_1aa60 : Constant  Value=Bva
  Constant_I_id_e8b3c : Constant  Value=I_id
  Constant_P_od_23920 : Constant  Value=P_od
  Constant_Vbase_a1dac : Constant  Value=Vbase
  Constant_Vdc_ref_dec2b : Constant  Value=Vdc_ref
  Constant_Vdcbase_412bc : Constant  Value=Vdcbase
  MathFunc_cos_8bffa : Trigonometry  Operator=cos
  MathFunc_sin_4068c : Trigonometry
  Product_2a033 : Product
  Product_30bc7 : Product
  Product_4f3af : Product
  Product_87d73 : Product
  Product_9b559 : Product
  Product_9e233 : Product
  Product_a81ab : Product
  Product_aa950 : Product
  Subtract_350a8 : Sum  Inputs=+-
  Subtract_5da16 : Sum  Inputs=+-
  Subtract_e9d84 : Sum  Inputs=+-
  Blockout_d_Phi_gb_GFL_17_572a8 : Outport
  wires:
  State_theta_pll_GFL_17_d7184/1 -> MathFunc_cos_8bffa/1
  MathFunc_cos_8bffa/1 -> Product_30bc7/2
  Constant_Bva_1aa60/1 -> Product_9b559/2
  State_theta_pll_GFL_17_d1250/1 -> MathFunc_sin_4068c/1
  Constant_-1_b59c1/1 -> Product_9b559/1
  Input_v_d_GFL_17_375e3/1 -> Product_30bc7/1
  Input_v_q_GFL_17_c3fa8/1 -> Product_a81ab/1
  MathFunc_sin_4068c/1 -> Product_a81ab/2
  Product_9b559/1 -> Product_87d73/1
  Constant_Vbase_a1dac/1 -> Product_87d73/2
  Product_30bc7/1 -> Subtract_350a8/1
  Product_a81ab/1 -> Subtract_350a8/2
  Constant_Vdc_ref_dec2b/1 -> Product_2a033/1
  Constant_Vdcbase_412bc/1 -> Product_2a033/2
  Product_87d73/1 -> Product_aa950/1
  Subtract_350a8/1 -> Product_aa950/2
  State_V_dc_GFL_17_71b96/1 -> Subtract_e9d84/1
  Constant_I_id_e8b3c/1 -> Product_4f3af/1
  Product_2a033/1 -> Subtract_e9d84/2
  Product_aa950/1 -> Add_c91bc/1
  State_Idv_GFL_17_5ec1c/1 -> Add_c91bc/2
  Constant_P_od_23920/1 -> Product_9e233/1
  Subtract_e9d84/1 -> Product_9e233/2
  Add_c91bc/1 -> Add_62c7f/1
  Product_9e233/1 -> Add_62c7f/2
  Add_62c7f/1 -> Add_0e360/1
  State_Phi_ga_GFL_17_0e94a/1 -> Add_0e360/2
  Add_0e360/1 -> Subtract_5da16/1
  State_i_gd_GFL_17_f44e4/1 -> Subtract_5da16/2
  Subtract_5da16/1 -> Product_4f3af/2
  Product_4f3af/1 -> Blockout_d_Phi_gb_GFL_17_572a8/1

== system IEEE14_case/GFL_17/d_Phi_gc_GFL_17_block ==
  note: d_Phi_gc_GFL_17 in case14gfl
      | $-I_{\mathrm{oq}}\,\left(\mathrm{Qe}_{\mathrm{ref}}\,\mathrm{Sbase}+1.73205080756888\,\mathrm{Vbase}\,i_{\mathrm{gd},\mathrm{GFL},17}\,\left(v_{q,\mathrm{GFL},17}\,\cos\left(\theta _{\mathrm{pll},\mathrm{GFL},17}\right)+v_{d,\mathrm{GFL},17}\,\sin\left(\theta _{\mathrm{pll},\mathrm{GFL},17}\right)\right)+1.73205080756888\,\mathrm{Vbase}\,i_{\mathrm{gq},\mathrm{GFL},17}\,\left(v_{d,\mathrm{GFL},17}\,\cos\left(\theta _{\mathrm{pll},\mathrm{GFL},17}\right)-v_{q,\mathrm{GFL},17}\,\sin\left(\theta _{\mathrm{pll},\mathrm{GFL},17}\right)\right)\right)$
      | Automatically generated on 2025-10-09 21:37:01 .
  State_i_gd_GFL_17_74615 : Inport
  Input_v_d_GFL_17_9c85a : Inport  Port=2
  State_theta_pll_GFL_17_39a31 : Inport  Port=3
  Input_v_q_GFL_17_9c131 : Inport  Port=4
  State_theta_pll_GFL_17_1661f : Inport  Port=5
  State_i_gq_GFL_17_83f75 : Inport  Port=6
  Input_v_d_GFL_17_ad008 : Inport  Port=7
  State_theta_pll_GFL_17_c6e4e : Inport  Port=8
  Input_v_q_GFL_17_b7629 : Inport  Port=9
  State_theta_pll_GFL_17_44558 : Inport  Port=10
  Add_616c7 : Sum
  Constant_-1_a9688 : Constant  Value=-1
  Constant_1.73205080756888_9db2c : Constant  Value=1.73205080756888
  Constant_1.73205080756888_ad4d1 : Constant  Value=1.73205080756888
  Constant_I_oq_2496f : Constant  Value=I_oq
  Constant_Qe_ref_1dd57 : Constant  Value=Qe_ref
  Constant_Sbase_edd80 : Constant  Value=Sbase
  Constant_Vbase_88f97 : Constant  Value=Vbase
  Constant_Vbase_f2aa4 : Constant  Value=Vbase
  MathFunc_cos_0de02 : Trigonometry  Operator=cos
  MathFunc_cos_65820 : Trigonometry  Operator=cos
  MathFunc_sin_0b4ae : Trigonometry
  MathFunc_sin_3e311 : Trigonometry
  Product_2148e : Product
  Product_22da6 : Product
  Product_2f214 : Product
  Product_3e297 : Product
  Product_45df5 : Product
  Product_4e2d5 : Product
  Product_64045 : Product
  Product_687de : Product
  Product_83e59 : Product
  Product_9dd55 : Product
  Product_c6d48 : Product
  Product_d555f : Product
  Product_ff510 : Product
  Subtract_15f60 : Sum  Inputs=+-
  Subtract_5a9e0 : Sum  Inputs=+-
  Subtract_dec6e : Sum  Inputs=+-
  Blockout_d_Phi_gc_GFL_17_224f3 : Outport
  wires:
  State_theta_pll_GFL_17_39a31/1 -> MathFunc_sin_3e311/1
  State_theta_pll_GFL_17_1661f/1 -> MathFunc_cos_65820/1
  Constant_Vbase_f2aa4/1 -> Product_64045/2
  Constant_Sbase_edd80/1 -> Product_9dd55/2
  Constant_1.73205080756888_ad4d1/1 -> Product_64045/1
  Input_v_d_GFL_17_9c85a/1 -> Product_d555f/1
  Constant_Qe_ref_1dd57/1 -> Product_45df5/2
  MathFunc_sin_3e311/1 -> Product_d555f/2
  Product_83e59/1 -> Add_616c7/2
  Input_v_q_GFL_17_9c131/1 -> Product_83e59/1
  MathFunc_cos_65820/1 -> Product_83e59/2
  State_theta_pll_GFL_17_c6e4e/1 -> MathFunc_cos_0de02/1
  MathFunc_sin_0b4ae/1 -> Product_22da6/2
  Constant_Vbase_88f97/1 -> Product_2f214/2
  State_theta_pll_GFL_17_44558/1 -> MathFunc_sin_0b4ae/1
  MathFunc_cos_0de02/1 -> Product_3e297/2
  Constant_-1_a9688/1 -> Product_45df5/1
  Product_64045/1 -> Product_687de/1
  State_i_gd_GFL_17_74615/1 -> Product_687de/2
  Product_d555f/1 -> Add_616c7/1
  Product_2f214/1 -> Product_2148e/1
  Constant_1.73205080756888_9db2c/1 -> Product_2f214/1
  Product_3e297/1 -> Subtract_dec6e/1
  Input_v_d_GFL_17_ad008/1 -> Product_3e297/1
  Product_22da6/1 -> Subtract_dec6e/2
  Product_45df5/1 -> Product_9dd55/1
  Input_v_q_GFL_17_b7629/1 -> Product_22da6/1
  Product_687de/1 -> Product_c6d48/1
  Add_616c7/1 -> Product_c6d48/2
  State_i_gq_GFL_17_83f75/1 -> Product_2148e/2
  Product_9dd55/1 -> Subtract_15f60/1
  Product_c6d48/1 -> Subtract_15f60/2
  Product_2148e/1 -> Product_4e2d5/1
  Subtract_dec6e/1 -> Product_4e2d5/2
  Subtract_15f60/1 -> Subtract_5a9e0/1
  Product_4e2d5/1 -> Subtract_5a9e0/2
  Constant_I_oq_2496f/1 -> Product_ff510/1
  Subtract_5a9e0/1 -> Product_ff510/2
  Product_ff510/1 -> Blockout_d_Phi_gc_GFL_17_224f3/1

== system IEEE14_case/GFL_17/d_Phi_gd_GFL_17_block ==
  note: d_Phi_gd_GFL_17 in case14gfl
      | $I_{\mathrm{iq}}\,\left(\mathrm{Iqv}_{\mathrm{GFL},17}+\Phi _{\mathrm{gc},\mathrm{GFL},17}-i_{\mathrm{gq},\mathrm{GFL},17}-P_{\mathrm{oq}}\,\left(\mathrm{Qe}_{\mathrm{ref}}\,\mathrm{Sbase}+1.73205080756888\,\mathrm{Vbase}\,i_{\mathrm{gd},\mathrm{GFL},17}\,\left(v_{q,\mathrm{GFL},17}\,\cos\left(\theta _{\mathrm{pll},\mathrm{GFL},17}\right)+v_{d,\mathrm{GFL},17}\,\sin\left(\theta _{\mathrm{pll},\mathrm{GFL},17}\right)\right)+1.73205080756888\,\mathrm{Vbase}\,i_{\mathrm{gq},\mathrm{GFL},17}\,\left(v_{d,\mathrm{GFL},17}\,\cos\left(\theta _{\mathrm{pll},\mathrm{GFL},17}\right)-v_{q,\mathrm{GFL},17}\,\sin\left(\theta _{\mathrm{pll},\mathrm{GFL},17}\right)\right)\right)+\mathrm{Bva}\,\mathrm{Vbase}\,\left(v_{q,\mathrm{GFL},17}\,\cos\left(\theta _{\mathrm{pll},\mathrm{GFL},17}\right)+v_{d,\mathrm{GFL},17}\,\sin\left(\theta _{\mathrm{pll},\mathrm{GFL},17}\right)\right)\right)$
      | Automatically generated on 2025-10-09 21:37:04 .
  Input_v_d_GFL_17_5111b : Inport
  State_theta_pll_GFL_17_b7930 : Inport  Port=2
  Input_v_q_GFL_17_e089c : Inport  Port=3
  State_theta_pll_GFL_17_4bbd3 : Inport  Port=4
  State_Iqv_GFL_17_1b144 : Inport  Port=5
  State_i_gd_GFL_17_cda7b : Inport  Port=6
  Input_v_d_GFL_17_2017d : Inport  Port=7
  State_theta_pll_GFL_17_40a47 : Inport  Port=8
  Input_v_q_GFL_17_bac0f : Inport  Port=9
  State_theta_pll_GFL_17_774b0 : Inport  Port=10
  State_i_gq_GFL_17_b900e : Inport  Port=11
  Input_v_d_GFL_17_a70b9 : Inport  Port=12
  State_theta_pll_GFL_17_735fc : Inport  Port=13
  Input_v_q_GFL_17_f280b : Inport  Port=14
  State_theta_pll_GFL_17_61b54 : Inport  Port=15
  State_Phi_gc_GFL_17_57f27 : Inport  Port=16
  State_i_gq_GFL_17_3bf40 : Inport  Port=17
  Add_339f1 : Sum
  Add_33b45 : Sum
  Add_bb697 : Sum
  Add_d09bb : Sum
  Add_edf24 : Sum
  Constant_-1_86e6d : Constant  Value=-1
  Constant_1.73205080756888_150ff : Constant  Value=1.73205080756888
  Constant_1.73205080756888_439a6 : Constant  Value=1.73205080756888
  Constant_Bva_027cc : Constant  Value=Bva
  Constant_I_iq_533d7 : Constant  Value=I_iq
  Constant_P_oq_c8b69 : Constant  Value=P_oq
  Constant_Qe_ref_6fe5e : Constant  Value=Qe_ref
  Constant_Sbase_62aa9 : Constant  Value=Sbase
  Constant_Vbase_16bd4 : Constant  Value=Vbase
  Constant_Vbase_60b4b : Constant  Value=Vbase
  Constant_Vbase_b798c : Constant  Value=Vbase
  MathFunc_cos_037db : Trigonometry  Operator=cos
  MathFunc_cos_5d9ec : Trigonometry  Operator=cos
  MathFunc_cos_f6076 : Trigonometry  Operator=cos
  MathFunc_sin_74c4d : Trigonometry
  MathFunc_sin_83fc7 : Trigonometry
  MathFunc_sin_e31d1 : Trigonometry
  Product_21129 : Product
  Product_2b728 : Product
  Product_2d541 : Product
  Product_3154a : Product
  Product_33515 : Product
  Product_428b0 : Product
  Product_64227 : Product
  Product_76a86 : Product
  Product_7b9c5 : Product
  Product_7c345 : Product
  Product_a1f07 : Product
  Product_a620f : Product
  Product_a70a3 : Product
  Product_b5077 : Product
  Product_bc700 : Product
  Product_c61e7 : Product
  Product_f36a8 : Product
  Product_f7cc8 : Product
  Subtract_a0b9c : Sum  Inputs=+-
  Subtract_d0e5f : Sum  Inputs=+-
  Subtract_e98a6 : Sum  Inputs=+-
  Subtract_ff8a9 : Sum  Inputs=+-
  Blockout_d_Phi_gd_GFL_17_94f94 : Outport
  wires:
  State_theta_pll_GFL_17_40a47/1 -> MathFunc_sin_74c4d/1
  MathFunc_sin_74c4d/1 -> Product_2b728/2
  State_theta_pll_GFL_17_774b0/1 -> MathFunc_cos_5d9ec/1
  Constant_Vbase_16bd4/1 -> Product_a1f07/2
  MathFunc_cos_5d9ec/1 -> Product_f7cc8/2
  Product_a1f07/1 -> Product_b5077/1
  Constant_1.73205080756888_439a6/1 -> Product_a1f07/1
  Product_2b728/1 -> Add_bb697/1
  Input_v_d_GFL_17_2017d/1 -> Product_2b728/1
  Input_v_q_GFL_17_bac0f/1 -> Product_f7cc8/1
  MathFunc_cos_037db/1 -> Product_428b0/2
  State_theta_pll_GFL_17_735fc/1 -> MathFunc_cos_037db/1
  Add_33b45/1 -> Add_d09bb/1
  State_i_gq_GFL_17_b900e/1 -> Product_64227/2
  State_theta_pll_GFL_17_61b54/1 -> MathFunc_sin_e31d1/1
  MathFunc_sin_83fc7/1 -> Product_a620f/2
  State_theta_pll_GFL_17_b7930/1 -> MathFunc_sin_83fc7/1
  Constant_Sbase_62aa9/1 -> Product_76a86/2
  State_theta_pll_GFL_17_4bbd3/1 -> MathFunc_cos_f6076/1
  Constant_-1_86e6d/1 -> Product_bc700/1
  MathFunc_cos_f6076/1 -> Product_a70a3/2
  Constant_Qe_ref_6fe5e/1 -> Product_bc700/2
  State_i_gd_GFL_17_cda7b/1 -> Product_b5077/2
  Product_f7cc8/1 -> Add_bb697/2
  Product_c61e7/1 -> Product_33515/1
  Constant_1.73205080756888_150ff/1 -> Product_f36a8/1
  MathFunc_sin_e31d1/1 -> Product_3154a/2
  Constant_Vbase_60b4b/1 -> Product_f36a8/2
  Input_v_d_GFL_17_a70b9/1 -> Product_428b0/1
  Input_v_q_GFL_17_f280b/1 -> Product_3154a/1
  Input_v_d_GFL_17_5111b/1 -> Product_a620f/1
  Input_v_q_GFL_17_e089c/1 -> Product_a70a3/1
  State_Iqv_GFL_17_1b144/1 -> Add_33b45/2
  Product_bc700/1 -> Product_76a86/1
  Product_b5077/1 -> Product_7b9c5/1
  Add_bb697/1 -> Product_7b9c5/2
  State_Phi_gc_GFL_17_57f27/1 -> Add_339f1/2
  Product_f36a8/1 -> Product_64227/1
  Product_33515/1 -> Add_33b45/1
  Product_428b0/1 -> Subtract_d0e5f/1
  Product_3154a/1 -> Subtract_d0e5f/2
  Constant_Bva_027cc/1 -> Product_c61e7/1
  Constant_Vbase_b798c/1 -> Product_c61e7/2
  Product_a620f/1 -> Add_edf24/1
  Product_a70a3/1 -> Add_edf24/2
  Product_76a86/1 -> Subtract_ff8a9/1
  Product_7b9c5/1 -> Subtract_ff8a9/2
  Product_64227/1 -> Product_21129/1
  Subtract_d0e5f/1 -> Product_21129/2
  Add_edf24/1 -> Product_33515/2
  Subtract_ff8a9/1 -> Subtract_e98a6/1
  Product_21129/1 -> Subtract_e98a6/2
  Constant_P_oq_c8b69/1 -> Product_7c345/1
  Subtract_e98a6/1 -> Product_7c345/2
  Product_7c345/1 -> Add_d09bb/2
  Add_d09bb/1 -> Add_339f1/1
  Product_2d541/1 -> Blockout_d_Phi_gd_GFL_17_94f94/1
  Add_339f1/1 -> Subtract_a0b9c/1
  State_i_gq_GFL_17_3bf40/1 -> Subtract_a0b9c/2
  Constant_I_iq_533d7/1 -> Product_2d541/1
  Subtract_a0b9c/1 -> Product_2d541/2

== system IEEE14_case/GFL_17/d_Phipll_GFL_17_block ==
  note: d_Phipll_GFL_17 in case14gfl
      | $-I_{\mathrm{pll}}\,\left(\mathrm{vq}_{\mathrm{ref}}+v_{q,\mathrm{GFL},17}\,\cos\left(\theta _{\mathrm{pll},\mathrm{GFL},17}\right)+v_{d,\mathrm{GFL},17}\,\sin\left(\theta _{\mathrm{pll},\mathrm{GFL},17}\right)\right)$
      | Automatically generated on 2025-10-09 21:36:55 .
  Input_v_d_GFL_17_09fe8 : Inport
  State_theta_pll_GFL_17_b324e : Inport  Port=2
  Input_v_q_GFL_17_cfbee : Inport  Port=3
  State_theta_pll_GFL_17_05e65 : Inport  Port=4
  Constant_-1_24f73 : Constant  Value=-1
  Constant_I_pll_fdfad : Constant  Value=I_pll
  Constant_vq_ref_f3995 : Constant  Value=vq_ref
  MathFunc_cos_ab3cc : Trigonometry  Operator=cos
  MathFunc_sin_9b72e : Trigonometry
  Product_1bb8e : Product
  Product_4990a : Product
  Product_580cd : Product
  Product_a6f96 : Product
  Subtract_9f158 : Sum  Inputs=+-
  Subtract_ca90c : Sum  Inputs=+-
  Blockout_d_Phipll_GFL_17_3d5a8 : Outport
  wires:
  State_theta_pll_GFL_17_05e65/1 -> MathFunc_cos_ab3cc/1
  Input_v_d_GFL_17_09fe8/1 -> Product_580cd/2
  Constant_-1_24f73/1 -> Product_580cd/1
  Input_v_q_GFL_17_cfbee/1 -> Product_1bb8e/1
  State_theta_pll_GFL_17_b324e/1 -> MathFunc_sin_9b72e/1
  Subtract_ca90c/1 -> Subtract_9f158/1
  Product_580cd/1 -> Product_4990a/1
  MathFunc_sin_9b72e/1 -> Product_4990a/2
  MathFunc_cos_ab3cc/1 -> Product_1bb8e/2
  Product_4990a/1 -> Subtract_ca90c/1
  Product_1bb8e/1 -> Subtract_ca90c/2
  Constant_vq_ref_f3995/1 -> Subtract_9f158/2
  Subtract_9f158/1 -> Product_a6f96/2
  Constant_I_pll_fdfad/1 -> Product_a6f96/1
  Product_a6f96/1 -> Blockout_d_Phipll_GFL_17_3d5a8/1

== system IEEE14_case/GFL_17/d_Psi_d_GFL_17_block ==
  note: d_Psi_d_GFL_17 in case14gfl
      | $-\frac{\Psi _{d,\mathrm{GFL},17}+\mathrm{Kdi}\,\mathrm{Vbase}\,\left(v_{q,\mathrm{GFL},17}\,\cos\left(\theta _{\mathrm{pll},\mathrm{GFL},17}\right)+v_{d,\mathrm{GFL},17}\,\sin\left(\theta _{\mathrm{pll},\mathrm{GFL},17}\right)\right)}{\mathrm{Tdi}}$
      | Automatically generated on 2025-10-09 21:37:06 .
  Input_v_d_GFL_17_e6869 : Inport
  State_theta_pll_GFL_17_99832 : Inport  Port=2
  Input_v_q_GFL_17_2c18f : Inport  Port=3
  State_theta_pll_GFL_17_a4bf5 : Inport  Port=4
  State_Psi_d_GFL_17_04c08 : Inport  Port=5
  Add_a0298 : Sum
  Constant_-1_0dece : Constant  Value=-1
  Constant_Kdi_4ec06 : Constant  Value=Kdi
  Constant_Tdi_2b38b : Constant  Value=Tdi
  Constant_Vbase_49200 : Constant  Value=Vbase
  Divide_5d26c : Product  Inputs=*/
  MathFunc_cos_eb5ff : Trigonometry  Operator=cos
  MathFunc_sin_d8b7b : Trigonometry
  Product_1172a : Product
  Product_ac690 : Product
  Product_d1d91 : Product
  Product_f5f9e : Product
  Product_fabe0 : Product
  Subtract_db9df : Sum  Inputs=+-
  Blockout_d_Psi_d_GFL_17_6e508 : Outport
  wires:
  State_theta_pll_GFL_17_a4bf5/1 -> MathFunc_cos_eb5ff/1
  MathFunc_sin_d8b7b/1 -> Product_d1d91/2
  MathFunc_cos_eb5ff/1 -> Product_f5f9e/2
  State_theta_pll_GFL_17_99832/1 -> MathFunc_sin_d8b7b/1
  Constant_-1_0dece/1 -> Product_fabe0/1
  Constant_Kdi_4ec06/1 -> Product_fabe0/2
  Input_v_d_GFL_17_e6869/1 -> Product_d1d91/1
  Input_v_q_GFL_17_2c18f/1 -> Product_f5f9e/1
  Product_fabe0/1 -> Product_ac690/1
  Constant_Vbase_49200/1 -> Product_ac690/2
  Product_d1d91/1 -> Add_a0298/1
  Product_f5f9e/1 -> Add_a0298/2
  Constant_Tdi_2b38b/1 -> Divide_5d26c/2
  Product_ac690/1 -> Product_1172a/1
  Add_a0298/1 -> Product_1172a/2
  Product_1172a/1 -> Subtract_db9df/1
  State_Psi_d_GFL_17_04c08/1 -> Subtract_db9df/2
  Subtract_db9df/1 -> Divide_5d26c/1
  Divide_5d26c/1 -> Blockout_d_Psi_d_GFL_17_6e508/1

== system IEEE14_case/GFL_17/d_Psi_q_GFL_17_block ==
  note: d_Psi_q_GFL_17 in case14gfl
      | $-\frac{\Psi _{q,\mathrm{GFL},17}-\mathrm{Kqi}\,\mathrm{Vbase}\,\left(v_{d,\mathrm{GFL},17}\,\cos\left(\theta _{\mathrm{pll},\mathrm{GFL},17}\right)-v_{q,\mathrm{GFL},17}\,\sin\left(\theta _{\mathrm{pll},\mathrm{GFL},17}\right)\right)}{\mathrm{Tqi}}$
      | Automatically generated on 2025-10-09 21:37:07 .
  Input_v_d_GFL_17_9db94 : Inport
  State_theta_pll_GFL_17_ec146 : Inport  Port=2
  Input_v_q_GFL_17_699cf : Inport  Port=3
  State_theta_pll_GFL_17_743ba : Inport  Port=4
  State_Psi_q_GFL_17_1cfcb : Inport  Port=5
  Constant_Kqi_ab3c7 : Constant  Value=Kqi
  Constant_Tqi_33ad0 : Constant  Value=Tqi
  Constant_Vbase_41cbc : Constant  Value=Vbase
  Divide_b6744 : Product  Inputs=*/
  MathFunc_cos_d58e9 : Trigonometry  Operator=cos
  MathFunc_sin_6fa67 : Trigonometry
  Product_56cf6 : Product
  Product_7043f : Product
  Product_98b8a : Product
  Product_a8fed : Product
  Subtract_c4e8e : Sum  Inputs=+-
  Subtract_e5c0d : Sum  Inputs=+-
  Blockout_d_Psi_q_GFL_17_9f89a : Outport
  wires:
  State_theta_pll_GFL_17_ec146/1 -> MathFunc_cos_d58e9/1
  State_Psi_q_GFL_17_1cfcb/1 -> Subtract_e5c0d/2
  State_theta_pll_GFL_17_743ba/1 -> MathFunc_sin_6fa67/1
  Input_v_d_GFL_17_9db94/1 -> Product_56cf6/1
  MathFunc_cos_d58e9/1 -> Product_56cf6/2
  Product_a8fed/1 -> Subtract_c4e8e/2
  Input_v_q_GFL_17_699cf/1 -> Product_a8fed/1
  Constant_Kqi_ab3c7/1 -> Product_98b8a/1
  MathFunc_sin_6fa67/1 -> Product_a8fed/2
  Constant_Vbase_41cbc/1 -> Product_98b8a/2
  Product_56cf6/1 -> Subtract_c4e8e/1
  Product_98b8a/1 -> Product_7043f/1
  Subtract_c4e8e/1 -> Product_7043f/2
  Product_7043f/1 -> Subtract_e5c0d/1
  Subtract_e5c0d/1 -> Divide_b6744/1
  Constant_Tqi_33ad0/1 -> Divide_b6744/2
  Divide_b6744/1 -> Blockout_d_Psi_q_GFL_17_9f89a/1
